simulink model "CurrentFunction"  (R2016a)
settings: Solver=VariableStepAuto  StartTime=0.0  StopTime=10.0  RelTol=1e-3
settings Model: Creator=enes_  LastModifiedBy=enes_

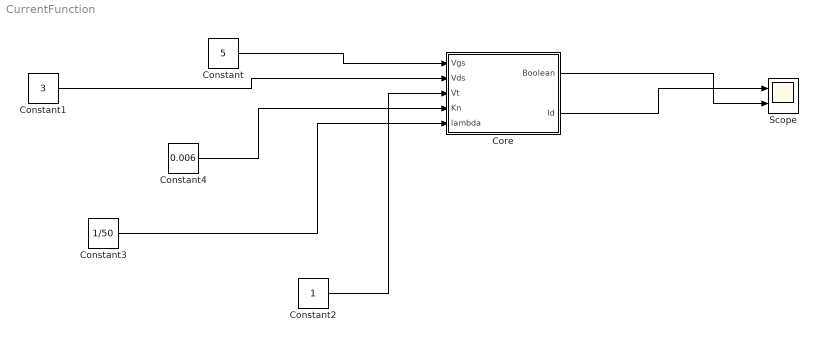
== system CurrentFunction ==
  Constant : Constant  Value=5
  Constant1 : Constant  Value=3
  Constant2 : Constant
  Constant3 : Constant  Value=1/50
  Constant4 : Constant  Value=0.006
  Core : Subsystem
  Scope : Scope  NumInputPorts=2
  wires:
  Core/2(Id) -> Scope/1
  Constant3/1 -> Core/5(lambda)
  Constant2/1 -> Core/3(Vt)
  Constant1/1 -> Core/2(Vds)
  Constant/1 -> Core/1(Vgs)
  Constant4/1 -> Core/4(Kn)
  Core/1(Boolean) -> Scope/2

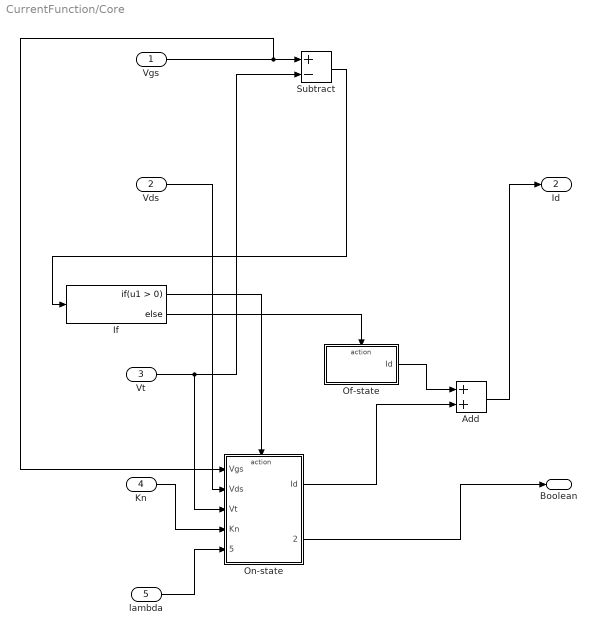
== system CurrentFunction/Core ==
  Vgs : Inport
  Vds : Inport  Port=2
  Vt : Inport  Port=3
  Kn : Inport  Port=4
  lambda : Inport  Port=5
  Add : Sum
  If : If
  Of-state : Subsystem  TreatAsAtomicUnit=on
  On-state : Subsystem  TreatAsAtomicUnit=on
  Subtract : Sum  Inputs=+-
  Boolean : Outport
  Id : Outport  Port=2
  wires:
  If/1 -> On-state/Action
  If/2 -> Of-state/Action
  Vt/1 -> On-state/3(Vt), Subtract/2
  Subtract/1 -> If/1
  Of-state/1(Id) -> Add/1
  On-state/1(Id) -> Add/2
  Add/1 -> Id/1
  On-state/2(Boolean) -> Boolean/1
  Kn/1 -> On-state/4(Kn)
  lambda/1 -> On-state/5(lambda)
  Vds/1 -> On-state/2(Vds)
  Vgs/1 -> On-state/1(Vgs), Subtract/1

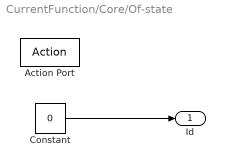
== system CurrentFunction/Core/Of-state ==
  Action Port : ActionPort  ActionType=else
  Constant : Constant  Value=0
  Id : Outport
  wires:
  Constant/1 -> Id/1

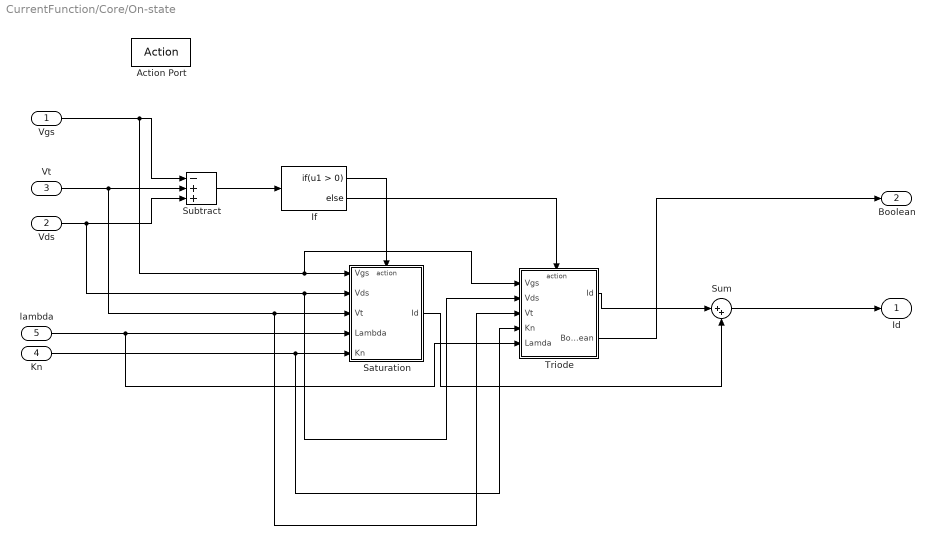
== system CurrentFunction/Core/On-state ==
  Vgs : Inport
  Vds : Inport  Port=2
  Vt : Inport  Port=3
  Kn : Inport  Port=4
  lambda : Inport  Port=5
  Action Port : ActionPort  ActionType=then
  If : If
  Saturation : Subsystem  TreatAsAtomicUnit=on
  Subtract : Sum  Inputs=-++
  Sum : Sum  Inputs=|++
  Triode : Subsystem  TreatAsAtomicUnit=on
  Id : Outport
  Boolean : Outport  Port=2
  wires:
  Vds/1 -> Triode/2(Vds), Saturation/2(Vds), Subtract/3
  Subtract/1 -> If/1
  If/1 -> Saturation/Action
  If/2 -> Triode/Action
  Vgs/1 -> Triode/1(Vgs), Saturation/1(Vgs), Subtract/1
  Vt/1 -> Triode/3(Vt), Saturation/3("Vt "), Subtract/2
  Kn/1 -> Triode/4(Kn), Saturation/5(Kn)
  lambda/1 -> Triode/5(Lamda), Saturation/4(Lambda)
  Triode/1(Id) -> Sum/1
  Saturation/1(Id) -> Sum/2
  Sum/1 -> Id/1
  Triode/2(Boolean) -> Boolean/1

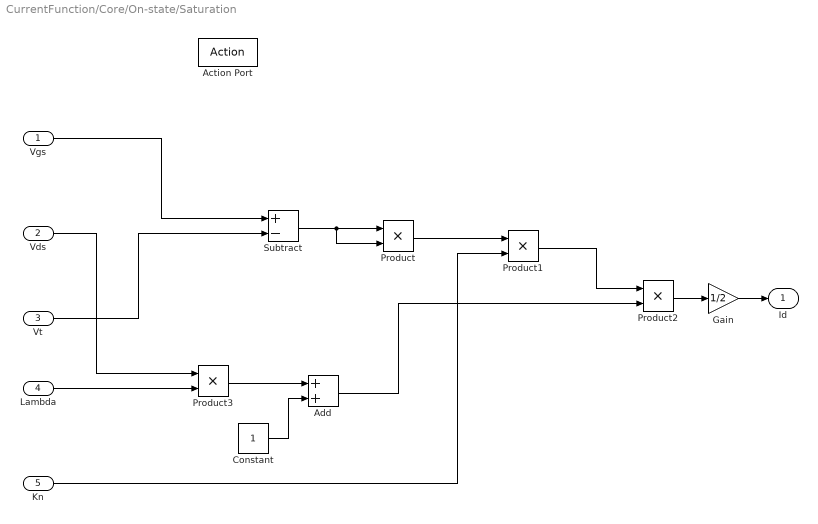
== system CurrentFunction/Core/On-state/Saturation ==
  Vgs : Inport
  Vds : Inport  Port=2
  "Vt " : Inport  Port=3
  Lambda : Inport  Port=4
  Kn : Inport  Port=5
  Action Port : ActionPort  ActionType=then
  Add : Sum
  Constant : Constant
  Gain : Gain  Gain=1/2
  Product{,1..3} (4 alike) : Product
  Subtract : Sum  Inputs=+-
  Id : Outport
  wires:
  Vgs/1 -> Subtract/1
  "Vt "/1 -> Subtract/2
  Subtract/1 -> Product/2, Product/1
  Kn/1 -> Product1/2
  Vds/1 -> Product3/1
  Lambda/1 -> Product3/2
  Product3/1 -> Add/1
  Constant/1 -> Add/2
  Add/1 -> Product2/2
  Product1/1 -> Product2/1
  Product2/1 -> Gain/1
  Product/1 -> Product1/1
  Gain/1 -> Id/1

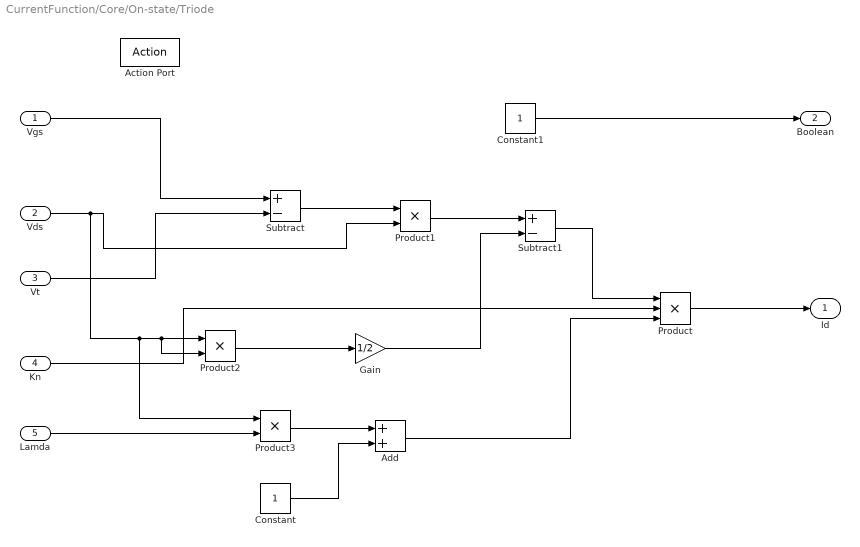
== system CurrentFunction/Core/On-state/Triode ==
  Vgs : Inport
  Vds : Inport  Port=2
  Vt : Inport  Port=3
  Kn : Inport  Port=4
  Lamda : Inport  Port=5
  Action Port : ActionPort  ActionType=else
  Add : Sum
  Constant : Constant
  Constant1 : Constant
  Gain : Gain  Gain=1/2
  Product : Product  Inputs=3
  Product1 : Product
  Product2 : Product
  Product3 : Product
  Subtract : Sum  Inputs=+-
  Subtract1 : Sum  Inputs=+-
  Id : Outport
  Boolean : Outport  Port=2
  wires:
  Vgs/1 -> Subtract/1
  Vt/1 -> Subtract/2
  Subtract/1 -> Product1/1
  Product1/1 -> Subtract1/1
  Product2/1 -> Gain/1
  Gain/1 -> Subtract1/2
  Vds/1 -> Product1/2, Product3/1, Product2/2, Product2/1
  Lamda/1 -> Product3/2
  Product3/1 -> Add/1
  Constant/1 -> Add/2
  Subtract1/1 -> Product/1
  Kn/1 -> Product/2
  Add/1 -> Product/3
  Product/1 -> Id/1
  Constant1/1 -> Boolean/1
